simulink model "model_problem1"  (R2020a)
settings: Solver=FixedStepAuto  StartTime=0.0  StopTime=10  RelTol=1e-3
values from neighbouring files (symbols this model uses):
  b = 50    [Initialisation.m]
  K1 = 50    [Initialisation.m]
  K12 = 1000    [Initialisation.m]
  M1 = 100    [Initialisation.m]
  M2 = 10    [Initialisation.m]
settings Model: Creator=Prateek  LastModifiedBy=Prateek

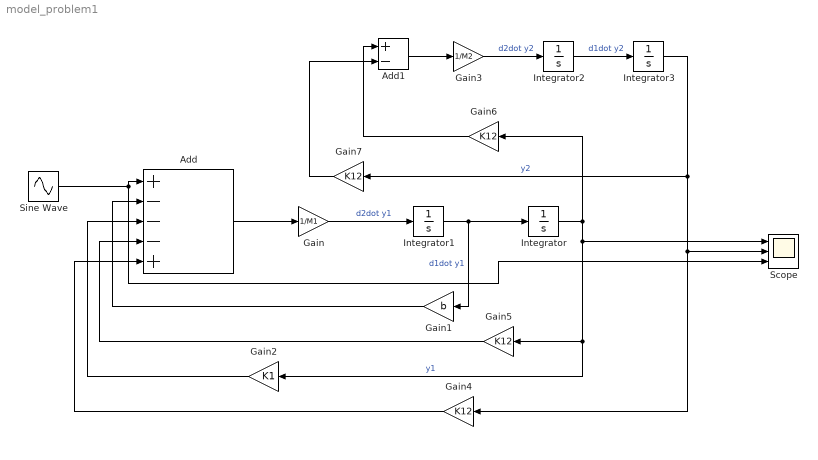
== system model_problem1 ==
  Add : Sum  Inputs=+---+
  Add1 : Sum  Inputs=+-
  Gain : Gain  Gain=1/M1
  Gain1 : Gain  Gain=b
  Gain2 : Gain  Gain=K1
  Gain3 : Gain  Gain=1/M2
  Gain{4..7} (4 alike) : Gain  Gain=K12
  Integrator{,1..3} (4 alike) : Integrator
  Scope : Scope  NumInputPorts=3
  Sine Wave : Sin  Amplitude=2  Frequency=10  SampleTime=0
  wires:
  Add/1 -> Gain/1
  Integrator/1 -> Gain6/1, Gain5/1, Gain2/1, Scope/1  "y1"
  Integrator2/1 -> Integrator3/1  "d1dot y2"
  Gain2/1 -> Add/3
  Add1/1 -> Gain3/1
  Integrator1/1 -> Gain1/1, Integrator/1  "d1dot y1"
  Gain3/1 -> Integrator2/1  "d2dot y2"
  Integrator3/1 -> Gain4/1, Scope/2, Gain7/1  "y2"
  Gain/1 -> Integrator1/1  "d2dot y1"
  Gain7/1 -> Add1/2
  Gain6/1 -> Add1/1
  Gain5/1 -> Add/4
  Sine Wave/1 -> Scope/3, Add/1
  Gain1/1 -> Add/2
  Gain4/1 -> Add/5
